simulink model "altitude_controller_design_harness"  (R2025b)
settings: Solver=VariableStepAuto  StartTime=0.0  StopTime=5  RelTol=1e-3
InitFcn:
  | currentControllerInit;
  | controller_mode = controller_modes.PRESSURE
  | 
  | fluid_constants;
  | plant_parameters;
undefined symbols (not defined in the file or in its folder): c_d, controller_modes, controllerGains, DiscIntNeverNeededParam, fluid, mass, nozzle_diameter, X0
libraries: simulink x7, metux_library x5, eeGeneralControl x4, simulink_extras x2, slpidlib x1
settings Model: DataDictionary=motorData.sldd  Creator=karadeli  LastModifiedBy=90507
settings DebuggingCC: ParamSuppressDoubleToSinglePrecisionLossMsg=on

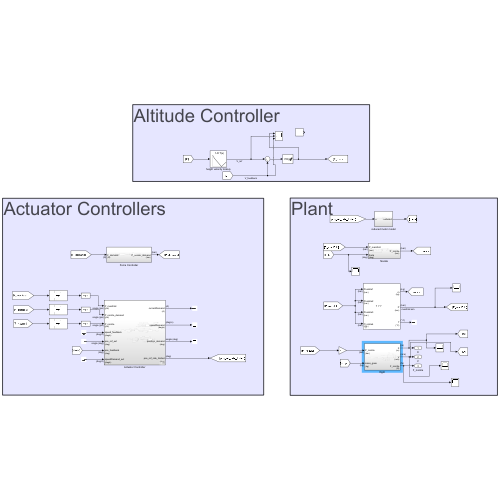
[thumbnail: Simulink's stored preview of the top-level diagram]
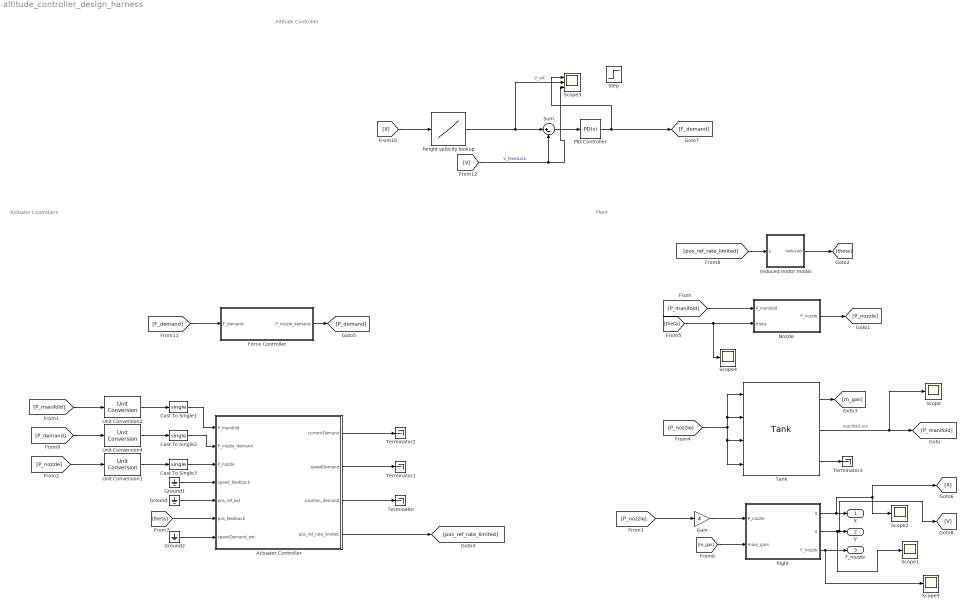
== system altitude_controller_design_harness ==
  note: Altitude Controller
  note: Actuator Controllers
  note: Plant
  Actuator Controller : Subsystem
  Cast To Single1 : DataTypeConversion  OutDataTypeStr=single  SaturateOnIntegerOverflow=off  RndMeth=Floor
  Cast To Single2 : DataTypeConversion  OutDataTypeStr=single  SaturateOnIntegerOverflow=off  RndMeth=Floor
  Cast To Single3 : DataTypeConversion  OutDataTypeStr=single  SaturateOnIntegerOverflow=off  RndMeth=Floor
  Force Controller : Subsystem
  Gain : Gain  Gain=4
  Ground : Ground
  Ground1 : Ground
  Ground2 : Ground
  Nozzle : Subsystem
  PID Controller : slpidlib/PID Controller  Controller=PD  Form=Parallel  TimeDomain=Continuous-time  UseExternalTs=off  SampleTime=-1  IntegratorMethod=Forward Euler  FilterMethod=Forward Euler  ControllerParametersSource=internal  P=180  I=1  UseKiTs=off  D=0  UseExternalDerivativeSource=off  N=100  UseFilter=on  TunerSelectOption=Transfer Function Based (PID Tuner App)  InitialConditionSource=internal  InitialConditionForIntegrator=0  InitialConditionForFilter=0  DifferentiatorICPrevScaledInput=0  ExternalReset=none  TrackingMode=off  Kt=1  LimitOutput=on  SatLimitsSource=internal  UpperSaturationLimit=inf  LowerSaturationLimit=0  LinearizeAsGain=on  AntiWindupMode=none  Kb=1  LimitIntegrator=off  UpperIntegratorSaturationLimit=inf  LowerIntegratorSaturationLimit=-inf  POutMin=[]  POutMax=[]  IOutMin=[]  IOutMax=[]  DOutMin=[]  DOutMax=[]  NOutMin=[]  NOutMax=[]  SumOutMin=[]  SumOutMax=[]  SaturationOutMin=[]  SaturationOutMax=[]  PParamMin=[]  PParamMax=[]  IParamMin=[]  IParamMax=[]  DParamMin=[]  DParamMax=[]  NParamMin=[]  NParamMax=[]  KbParamMin=[]  KbParamMax=[]  KtParamMin=[]  KtParamMax=[]  KbOutMin=[]  KbOutMax=[]  KtOutMin=[]  KtOutMax=[]  IntegratorOutMin=[]  IntegratorOutMax=[]  FilterOutMin=[]  FilterOutMax=[]  SumI1OutMin=[]  SumI1OutMax=[]  SumI2OutMin=[]  SumI2OutMax=[]  SumI3OutMin=[]  SumI3OutMax=[]  SumI4OutMin=[]  SumI4OutMax=[]  SumDOutMin=[]  SumDOutMax=[]  DifferentiatorOutMin=[]  DifferentiatorOutMax=[]  FilterDiffOutCoefMin=[]  FilterDiffOutCoefMax=[]  ReciprocalOutMin=[]  ReciprocalOutMax=[]  SumDenOutMin=[]  SumDenOutMax=[]  SumNumOutMin=[]  SumNumOutMax=[]  DivideOutMin=[]  DivideOutMax=[]  UdiffTsProdOutMin=[]  UdiffTsProdOutMax=[]  NTsProdOutMin=[]  NTsProdOutMax=[]  UintegralTsProdOutMin=[]  UintegralTsProdOutMax=[]  UngainTsProdOutMin=[]  UngainTsProdOutMax=[]  ClampingZeroOutDataTypeStr=Inherit: Inherit via back propagation  ClampingZeroOutMin=[]  ClampingZeroOutMax=[]  FilterDenConstantOutDataTypeStr=Inherit: Inherit via back propagation  FilterDenConstantOutMin=[]  FilterDenConstantOutMax=[]  PCopyOutDataTypeStr=Inherit: Inherit via back propagation  PCopyOutMin=[]  PCopyOutMax=[]  NCopyOutDataTypeStr=Inherit: Inherit via back propagation  NCopyOutMin=[]  NCopyOutMax=[]  IntegratorContinuousStateAttributes=''  IntegratorStateMustResolveToSignalObject=off  IntegratorRTWStateStorageClass=Auto  FilterContinuousStateAttributes=''  FilterStateMustResolveToSignalObject=off  FilterRTWStateStorageClass=Auto  ParallelPVariant=InternalParameters  IdealPVariant=Disabled  IVariant=Disabled  DVariant=InternalParameters  IntegratorVariant=Disabled  SatVariant=Enabled  AWVariant=Disabled  PCopyVariant=Disabled  TRVariant=Disabled  FdbkBlocksVariant=Forward  IdealPFdbkVariant=Disabled  SatFdbkVariant=Disabled  DerivativeFilterVariant=ContFilter  NVariant=InternalParameters  NCopyVariant=Disabled  FilterICVariant=InternalICsFilter  IntegratorICVariant=Disabled  ExternalResetVariant=Disabled  TRSumVariant=Passthrough  SumFdbkVariant=Disabled  SumVariant=Sum_PD  TsampFilterVariant=InternalTs  TsampNgainVariant=Passthrough  TsampIntegralVariant=Disabled_SignalSpec  ExternalSaturationOutDataTypeStr=Inherit: Same as second input  DerivativeSourceVariant=ErrorSignal  PreIntVariant=InternalPreInt
  Scope{,1..2,4..5} (5 alike) : Scope
      Scope settings: ActiveDisplayYMinimum=-1  ActiveDisplayYMaximum=1  DataLoggingVariableName=ScopeData12
      Scope1 settings: ActiveDisplayYMinimum=-12.245566347072526  ActiveDisplayYMaximum=6.6093021776689689  DataLoggingVariableName=ScopeData13
      Scope2 settings: ActiveDisplayYMinimum=-1.1324371537865316  ActiveDisplayYMaximum=10.125826350420725  DataLoggingVariableName=ScopeData14
      Scope4 settings: ActiveDisplayYMinimum=-135.02216749767223  ActiveDisplayYMaximum=1215.1995074790502  DataLoggingVariableName=ScopeData24
      Scope5 settings: ActiveDisplayYMinimum=-1  ActiveDisplayYMaximum=1  DataLoggingVariableName=ScopeData25
  Scope3 : Scope  NumInputPorts=3
      settings: ActiveDisplayYMinimum=-1  ActiveDisplayYMaximum=1  DataLoggingVariableName=ScopeData15
  Step : Step  Time=0.75  After=180  SampleTime=0
  Sum : Sum  Inputs=|+-
  Tank : metux_library/Tank  P0=300  T0=40  mdotGain=fluid.mdotGain  V=fluid.V  R=fluid.R  Cv=fluid.Cv  Patm=fluid.Patm
  Terminator{,1..3} (4 alike) : Terminator
  Unit Conversion1 : UnitConversion
  Unit Conversion2 : UnitConversion
  Unit Conversion4 : UnitConversion
  flight : Subsystem
  height velocity lookup : Lookup_n-D  NumberOfTableDimensions=1  BreakpointsForDimension1=[0 1 6 9]  Table=[0 -2 -8 -5]  InternalRulePriority=Speed  RndMeth=Simplest
  reduced motor model : Subsystem
  X : Outport
  V : Outport  Port=2
  F_nozzle : Outport  Port=3
  wires:
  flight/2(V) -> Scope1/1, [V], V/1
  flight/3(F_nozzle) -> Scope5/1, F_nozzle/1
  flight/1(X) -> [X], Scope2/1, X/1
  [theta] -> Scope4/1, Nozzle/2(theta)
  Tank/2 -> [P_manifold], Scope/1  "manifold sim"
  [P_manifold] -> Unit Conversion2/1
  Actuator Controller/3(position_demand) -> Terminator/1
  Actuator Controller/2(speedDemand) -> Terminator1/1
  Actuator Controller/1(currentDemand) -> Terminator2/1
  Ground/1 -> Actuator Controller/5(pos_ref_ext)
  Tank/1 -> [m_gas]
  [m_gas] -> flight/2(mass_gass)
  Tank/3 -> Terminator3/1
  reduced motor model/1(reduced) -> [theta]
  [theta] -> Actuator Controller/6(pos_feedback)
  [pos_ref_rate_limited] -> reduced motor model/1(u)
  Cast To Single2/1 -> Actuator Controller/2(P_nozzle_demand)
  Ground1/1 -> Actuator Controller/4(speed_feedback)
  Ground2/1 -> Actuator Controller/7(speedDemand_ext)
  [P_nozzle] -> Tank/1, Tank/2, Tank/4, Tank/3
  Nozzle/1(P_nozzle) -> [P_nozzle]
  Unit Conversion4/1 -> Cast To Single2/1
  [P_manifold] -> Nozzle/1(P_manifold)
  Unit Conversion1/1 -> Cast To Single3/1
  [P_nozzle] -> Gain/1
  [P_nozzle] -> Unit Conversion1/1
  Cast To Single3/1 -> Actuator Controller/3(P_nozzle)
  Unit Conversion2/1 -> Cast To Single1/1
  Cast To Single1/1 -> Actuator Controller/1(P_manifold)
  Force Controller/1(P_nozzle_demand) -> [P_demand]
  [P_demand] -> Unit Conversion4/1
  Actuator Controller/4(pos_ref_rate_limited) -> [pos_ref_rate_limited]
  Sum/1 -> PID Controller/1
  PID Controller/1 -> Scope3/1, [F_demand]
  [F_demand] -> Force Controller/1(F_demand)
  height velocity lookup/1 -> Scope3/2, Sum/1  "V_ref"
  [X] -> height velocity lookup/1
  [V] -> Scope3/3, Sum/2  "V_feedback"
  Gain/1 -> flight/1(P_nozzle)

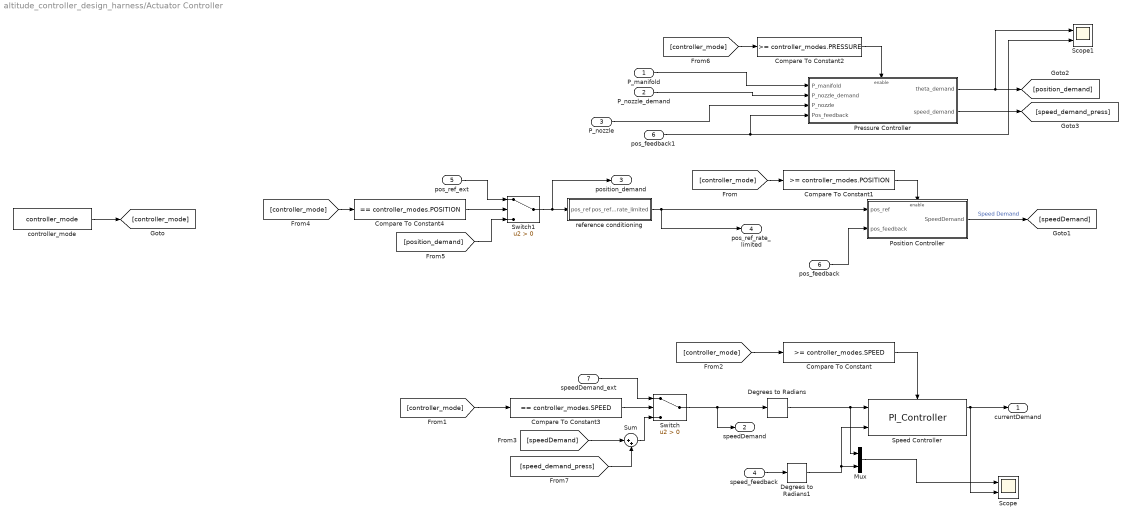
== system altitude_controller_design_harness/Actuator Controller ==
  P_manifold : Inport  OutDataTypeStr=single  Unit=psi  PortDimensions=1  SampleTime=1/1000
  P_nozzle_demand : Inport  Port=2  OutDataTypeStr=single  Unit=psi  PortDimensions=1  SampleTime=1/1000
  P_nozzle : Inport  Port=3  OutDataTypeStr=single  Unit=psi  PortDimensions=1  SampleTime=1/1000
  speed_feedback : Inport  Port=4  Unit=deg/s  SampleTime=controllerGains.speed.Ts  Interpolate=off
  pos_ref_ext : Inport  Port=5  OutDataTypeStr=single  Unit=deg  SampleTime=controllerGains.position.Ts  Interpolate=off
  pos_feedback : Inport  Port=6  Unit=deg  SampleTime=controllerGains.position.Ts  Interpolate=off
  speedDemand_ext : Inport  Port=7  Unit=deg/s
  Compare To Constant : simulink/Logic and Bit Operations/Compare To Constant  relop=>=  const=controller_modes.SPEED  OutDataTypeStr=boolean
  Compare To Constant1 : simulink/Logic and Bit Operations/Compare To Constant  relop=>=  const=controller_modes.POSITION  OutDataTypeStr=boolean
  Compare To Constant2 : simulink/Logic and Bit Operations/Compare To Constant  relop=>=  const=controller_modes.PRESSURE  OutDataTypeStr=boolean
  Compare To Constant3 : simulink/Logic and Bit Operations/Compare To Constant  relop===  const=controller_modes.SPEED  OutDataTypeStr=boolean
  Compare To Constant4 : simulink/Logic and Bit Operations/Compare To Constant  relop===  const=controller_modes.POSITION  OutDataTypeStr=boolean
  Degrees to Radians : simulink_extras/Transformations/Degrees to Radians
  Degrees to Radians1 : simulink_extras/Transformations/Degrees to Radians
  Mux : Mux  Inputs=2
  Position Controller : Subsystem
  Pressure Controller : Subsystem
  Scope : Scope  NumInputPorts=2
      settings: ActiveDisplayYMinimum=-3482.2818450927725  ActiveDisplayYMaximum=28164.697982788086
  Scope1 : Scope  NumInputPorts=2
      settings: ActiveDisplayYMinimum=-329.76221466064453  ActiveDisplayYMaximum=370.11640167236328
  Speed Controller : metux_library/PI_Controller  Kp=controllerGains.speed.Kp  Ki=controllerGains.speed.Ki  SatMax=controllerGains.speed.SatMax  SatMin=controllerGains.speed.SatMin  Ts=controllerGains.speed.Ts  RateLimiterMax=controllerGains.speed.RateLimiterMax  RateLimiterMin=controllerGains.speed.RateLimiterMin
  Sum : Sum  Inputs=|++
  Switch : Switch  Criteria=u2 > Threshold  SaturateOnIntegerOverflow=off  InputSameDT=off
  Switch1 : Switch  Criteria=u2 > Threshold  SaturateOnIntegerOverflow=off  InputSameDT=off
  controller_mode : Constant  Value=controller_mode  SampleTime=-1
  pos_feedback1 : InportShadow  Port=6  Unit=deg  SampleTime=controllerGains.position.Ts  Interpolate=off
  reference conditioning : Subsystem
  currentDemand : Outport  Unit=A
  speedDemand : Outport  Port=2  Unit=deg/s
  position_demand : Outport  Port=3  OutDataTypeStr=single  Unit=deg
  pos_ref_rate_limited : Outport  Port=4  Unit=deg  SampleTime=1/1000
  wires:
  Pressure Controller/1(theta_demand) -> [position_demand], Scope1/1
  P_nozzle_demand/1 -> Pressure Controller/2(P_nozzle_demand)
  [controller_mode] -> Compare To Constant4/1
  controller_mode/1 -> [controller_mode]
  speedDemand_ext/1 -> Switch/1
  Mux/1 -> Scope/1
  Sum/1 -> Switch/3
  speed_feedback/1 -> Degrees to Radians1/1
  Position Controller/1(SpeedDemand) -> [speedDemand]  "Speed Demand"
  Degrees to Radians/1 -> Mux/1, Speed Controller/1
  Switch/1 -> speedDemand/1, Degrees to Radians/1
  Compare To Constant1/1 -> Position Controller/Enable
  [controller_mode] -> Compare To Constant2/1
  Compare To Constant/1 -> Speed Controller/Enable
  pos_feedback/1 -> Position Controller/2(pos_feedback)
  Compare To Constant2/1 -> Pressure Controller/Enable
  P_nozzle/1 -> Pressure Controller/3(P_nozzle)
  Compare To Constant4/1 -> Switch1/2
  [position_demand] -> Switch1/3
  [controller_mode] -> Compare To Constant1/1
  Speed Controller/1 -> currentDemand/1, Scope/2
  [controller_mode] -> Compare To Constant/1
  P_manifold/1 -> Pressure Controller/1(P_manifold)
  pos_ref_ext/1 -> Switch1/1
  Switch1/1 -> position_demand/1, reference conditioning/1(pos_ref)
  Degrees to Radians1/1 -> Speed Controller/2, Mux/2
  [controller_mode] -> Compare To Constant3/1
  Compare To Constant3/1 -> Switch/2
  reference conditioning/1(pos_ref_rate_limited) -> pos_ref_rate_limited/1, Position Controller/1(pos_ref)
  pos_feedback1/1 -> Pressure Controller/4(Pos_feedback), Scope1/2
  Pressure Controller/2(speed_demand) -> [speed_demand_press]
  [speedDemand] -> Sum/1
  [speed_demand_press] -> Sum/2

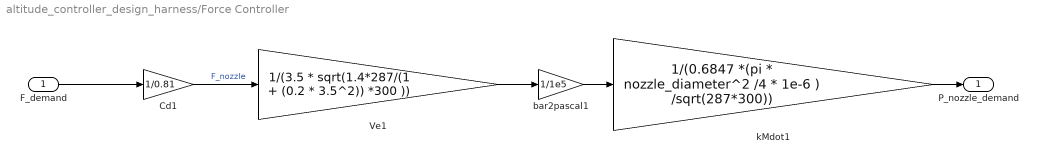
== system altitude_controller_design_harness/Force Controller ==
  F_demand : Inport  Unit=N  SampleTime=1/1000
  Cd1 : Gain  Gain=1/0.81
  Ve1 : Gain  Gain=1/(3.5 * sqrt(1.4*287/(1 + (0.2 * 3.5^2)) *300 ))
  bar2pascal1 : Gain  Gain=1/1e5
  kMdot1 : Gain  Gain=1/(0.6847 *(pi * nozzle_diameter^2 /4 * 1e-6 ) /sqrt(287*300))
  P_nozzle_demand : Outport  Unit=bar  SampleTime=1/1000
  wires:
  kMdot1/1 -> P_nozzle_demand/1
  bar2pascal1/1 -> kMdot1/1
  Ve1/1 -> bar2pascal1/1
  Cd1/1 -> Ve1/1  "F_nozzle"
  F_demand/1 -> Cd1/1

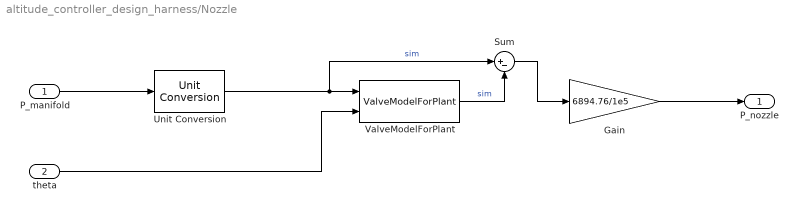
== system altitude_controller_design_harness/Nozzle ==
  P_manifold : Inport  Unit=bar
  theta : Inport  Port=2  Unit=deg
  Gain : Gain  Gain=6894.76/1e5
  Sum : Sum  Inputs=|+-
  Unit Conversion : UnitConversion
  ValveModelForPlant : metux_library/ValveModelForPlant  C_max=0.9197  alpha=51.8534
  P_nozzle : Outport  Unit=bar
  wires:
  theta/1 -> ValveModelForPlant/2
  P_manifold/1 -> Unit Conversion/1
  Sum/1 -> Gain/1
  ValveModelForPlant/1 -> Sum/2  "sim"
  Gain/1 -> P_nozzle/1
  Unit Conversion/1 -> Sum/1, ValveModelForPlant/1  "sim"

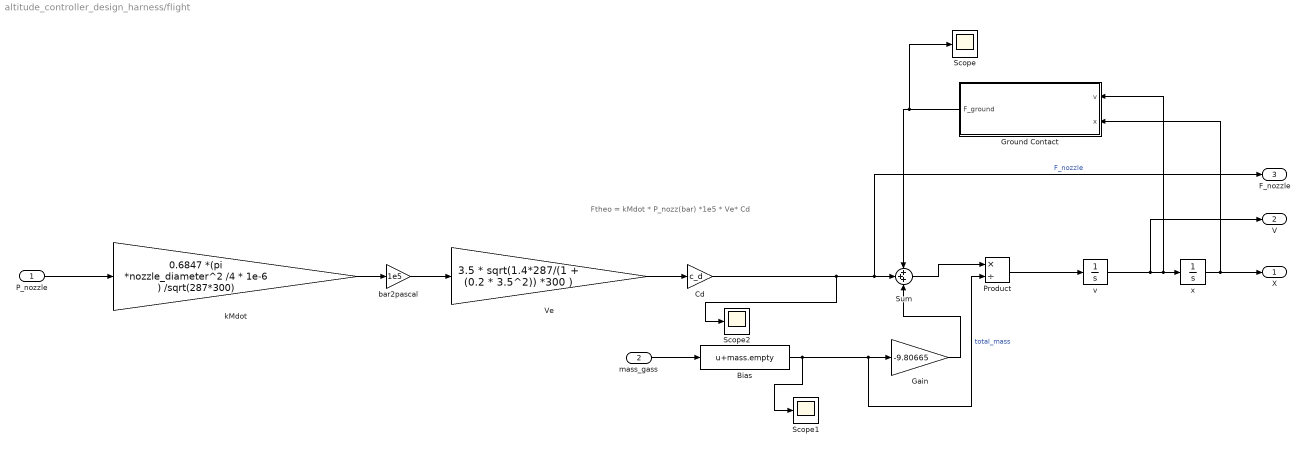
== system altitude_controller_design_harness/flight ==
  note: Ftheo = kMdot * P_nozz(bar) *1e5 * Ve* Cd
  P_nozzle : Inport  Unit=bar
  mass_gass : Inport  Port=2  Unit=kg
  Bias : Bias  Bias=mass.empty  SaturateOnIntegerOverflow=off
  Cd : Gain  Gain=c_d
  Gain : Gain  Gain=-9.80665
  Ground Contact : Subsystem
  Product : Product  Inputs=*/
  Scope : Scope
      settings: ActiveDisplayYMinimum=-179.96473711218755  ActiveDisplayYMaximum=786.35837452552653  DataLoggingVariableName=ScopeData19
  Scope1 : Scope
      settings: ActiveDisplayYMinimum=-1  ActiveDisplayYMaximum=1  DataLoggingVariableName=ScopeData20
  Scope2 : Scope
      settings: ActiveDisplayYMinimum=-1  ActiveDisplayYMaximum=1  DataLoggingVariableName=ScopeData21
  Sum : Sum  Inputs=+++
  Ve : Gain  Gain=3.5 * sqrt(1.4*287/(1 + (0.2 * 3.5^2)) *300 )
  bar2pascal : Gain  Gain=1e5
  kMdot : Gain  Gain=0.6847 *(pi *nozzle_diameter^2 /4 * 1e-6 ) /sqrt(287*300)
  v : Integrator
  x : Integrator  InitialCondition=X0
  X : Outport  Unit=m
  V : Outport  Port=2  Unit=m/s
  F_nozzle : Outport  Port=3  Unit=N
  wires:
  Gain/1 -> Sum/3
  Sum/1 -> Product/1
  x/1 -> Ground Contact/2(x), X/1
  kMdot/1 -> bar2pascal/1
  Bias/1 -> Scope1/1, Product/2, Gain/1  "total_mass"
  bar2pascal/1 -> Ve/1
  Cd/1 -> Scope2/1, F_nozzle/1, Sum/2  "F_nozzle"
  Product/1 -> v/1
  Ve/1 -> Cd/1
  P_nozzle/1 -> kMdot/1
  mass_gass/1 -> Bias/1
  v/1 -> Ground Contact/1(v), x/1, V/1
  Ground Contact/1(F_ground) -> Scope/1, Sum/1

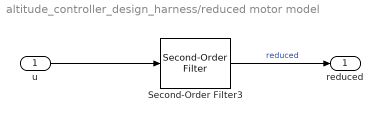
== system altitude_controller_design_harness/reduced motor model ==
  u : Inport
  Second-Order Filter3 : eeGeneralControl/Second-Order Filter  FilterType=Low-pass  fn=21.64  Zeta=0.86  Ts=-1  A0=0  Ph0=0  f0=0  b0=0
      settings: LibrarySourceBlock=ee_sl_lib/General Control/Second-Order Filter
  reduced : Outport
  wires:
  Second-Order Filter3/1 -> reduced/1  "reduced"
  u/1 -> Second-Order Filter3/1

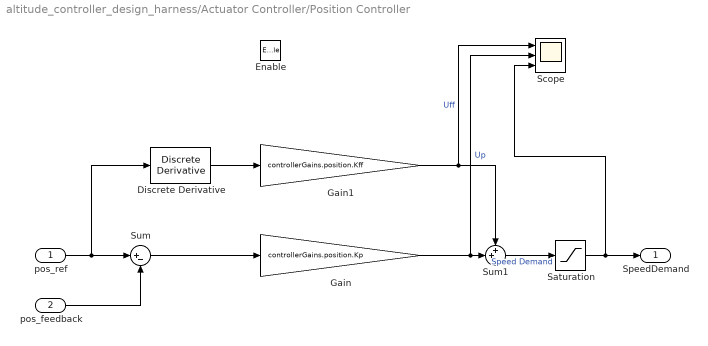
== system altitude_controller_design_harness/Actuator Controller/Position Controller ==
  pos_ref : Inport  Unit=deg
  pos_feedback : Inport  Port=2  Unit=deg
  Enable : EnablePort  StatesWhenEnabling=reset
  Discrete Derivative : simulink/Discrete/Discrete Derivative  gainval=1.0  ICPrevScaledInput=0.0  OutMin=[]  OutMax=[]  OutDataType=fixdt(1, 16)  OutScaling=2^-10  DoSatur=off
  Gain : Gain  Gain=controllerGains.position.Kp
  Gain1 : Gain  Gain=controllerGains.position.Kff
  Saturation : Saturate  UpperLimit=controllerGains.position.SatMax  LowerLimit=controllerGains.position.SatMin
  Scope : Scope  NumInputPorts=3
      settings: ActiveDisplayYMinimum=-3294.8933715820312  ActiveDisplayYMaximum=3471.4622192382812
  Sum : Sum  Inputs=|+-
  Sum1 : Sum  Inputs=++|
  SpeedDemand : Outport  Unit=deg/s  OutputWhenDisabled=reset  InitialOutput=[0.0]
  wires:
  Saturation/1 -> Scope/3, SpeedDemand/1
  pos_feedback/1 -> Sum/2
  Gain/1 -> Scope/2, Sum1/2  "Up"
  Sum/1 -> Gain/1
  pos_ref/1 -> Discrete Derivative/1, Sum/1
  Sum1/1 -> Saturation/1  "Speed Demand"
  Discrete Derivative/1 -> Gain1/1
  Gain1/1 -> Scope/1, Sum1/1  "Uff"

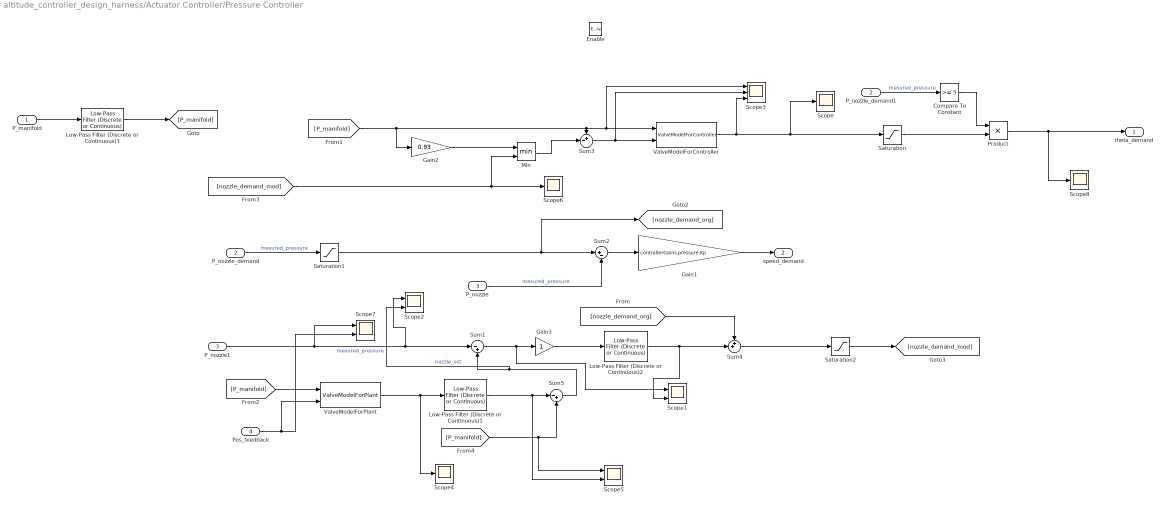
== system altitude_controller_design_harness/Actuator Controller/Pressure Controller ==
  P_manifold : Inport
  P_nozzle_demand : Inport  Port=2
  P_nozzle : Inport  Port=3
  Pos_feedback : Inport  Port=4
  Enable : EnablePort  StatesWhenEnabling=reset
  Compare To Constant : simulink/Logic and Bit Operations/Compare To Constant  relop=>=  const=5  OutDataTypeStr=boolean
  Gain1 : Gain  Gain=controllerGains.pressure.Kp
  Gain2 : Gain  Gain=0.93
  Gain3 : Gain
  Low-Pass Filter (Discrete or Continuous)1 : eeGeneralControl/Low-Pass Filter (Discrete or Continuous)  K=1  T=0.001  B=inf  A=-inf  init_option=Inherited from block input  x0=0  Ts=-1
  Low-Pass Filter (Discrete or Continuous)2 : eeGeneralControl/Low-Pass Filter (Discrete or Continuous)  K=1  T=0.004  B=250  A=-250  init_option=Inherited from block input  x0=0  Ts=-1
  Low-Pass Filter (Discrete or Continuous)3 : eeGeneralControl/Low-Pass Filter (Discrete or Continuous)  K=single(1)  T=single(0.005)  B=inf  A=-inf  init_option=Inherited from block input  x0=0  Ts=-1
  Min : MinMax  Inputs=2
  P_nozzle1 : InportShadow  Port=3
  P_nozzle_demand1 : InportShadow  Port=2
  Product : Product
  Saturation : Saturate  UpperLimit=1080  LowerLimit=0
  Saturation1 : Saturate  UpperLimit=4000  LowerLimit=0
  Saturation2 : Saturate  UpperLimit=4000  LowerLimit=0
  Scope{,4,6,8} (4 alike) : Scope
      Scope settings: ActiveDisplayYMinimum=-15.395192146301266  ActiveDisplayYMaximum=138.55672931671143  DataLoggingVariableName=ScopeData2
      Scope4 settings: ActiveDisplayYMinimum=1007.1971893310547  ActiveDisplayYMaximum=2357.6605987548828  DataLoggingVariableName=ScopeData6
      Scope6 settings: ActiveDisplayYMinimum=-112.49999999999997  ActiveDisplayYMaximum=1012.5  DataLoggingVariableName=ScopeData8
      Scope8 settings: ActiveDisplayYMinimum=-18.167575836181637  ActiveDisplayYMaximum=163.50818252563477  DataLoggingVariableName=ScopeData10
  Scope{1..2,5,7} (4 alike) : Scope  NumInputPorts=2
      Scope1 settings: ActiveDisplayYMinimum=16.466037750244148  ActiveDisplayYMaximum=359.39812850952148  DataLoggingVariableName=ScopeData4
      Scope2 settings: ActiveDisplayYMinimum=-179.26073789596555  ActiveDisplayYMaximum=1025.8466792106628  DataLoggingVariableName=ScopeData5
      Scope5 settings: ActiveDisplayYMinimum=1218.2213745117188  ActiveDisplayYMaximum=2587.3870239257812  DataLoggingVariableName=ScopeData7
      Scope7 settings: ActiveDisplayYMinimum=-62.757351875305176  ActiveDisplayYMaximum=64.080883979797363  DataLoggingVariableName=ScopeData9
  Scope3 : Scope  NumInputPorts=3
      settings: ActiveDisplayYMinimum=-431.94372558593739  ActiveDisplayYMaximum=3887.4935302734375  DataLoggingVariableName=ScopeData3
  Sum1 : Sum  Inputs=|-+
  Sum2 : Sum  Inputs=|+-
  Sum3 : Sum  Inputs=+-|  OutDataTypeStr=single
  Sum4 : Sum  Inputs=++|
  Sum5 : Sum  Inputs=|-+
  ValveModelForController : metux_library/ValveModelForController  alpha=51.8534  C_max=0.9197
  ValveModelForPlant : metux_library/ValveModelForPlant  C_max=0.9197  alpha=51.8534
  theta_demand : Outport  OutputWhenDisabled=reset  InitialOutput=0
  speed_demand : Outport  Port=2  OutputWhenDisabled=reset  InitialOutput=0
  wires:
  Saturation/1 -> Product/2
  Compare To Constant/1 -> Product/1
  P_nozzle_demand1/1 -> Compare To Constant/1  "mesured_pressure"
  Saturation2/1 -> [nozzle_demand_mod]
  Saturation1/1 -> [nozzle_demand_org], Sum2/1
  Sum1/1 -> Gain3/1, Scope1/1
  Product/1 -> theta_demand/1, Scope8/1
  Gain2/1 -> Min/1
  P_manifold/1 -> Low-Pass Filter (Discrete or Continuous)3/1
  P_nozzle_demand/1 -> Saturation1/1  "mesured_pressure"
  Sum3/1 -> Scope3/2, ValveModelForController/2
  P_nozzle/1 -> Sum2/2  "mesured_pressure"
  Gain1/1 -> speed_demand/1
  ValveModelForController/1 -> Scope3/3, Saturation/1, Scope/1
  Sum2/1 -> Gain1/1
  ValveModelForPlant/1 -> Low-Pass Filter (Discrete or Continuous)1/1, Scope4/1
  Sum5/1 -> Sum1/2, Scope2/2  "nozzle_est"
  [nozzle_demand_org] -> Sum4/1
  [P_manifold] -> Sum5/2, Scope5/1
  Sum4/1 -> Saturation2/1
  [nozzle_demand_mod] -> Scope6/1, Min/2
  Min/1 -> Sum3/2
  Gain3/1 -> Low-Pass Filter (Discrete or Continuous)2/1
  Pos_feedback/1 -> ValveModelForPlant/2, Scope7/2
  [P_manifold] -> ValveModelForPlant/1
  [P_manifold] -> Sum3/1, Scope3/1, ValveModelForController/1, Gain2/1
  Low-Pass Filter (Discrete or Continuous)1/1 -> Sum5/1, Scope5/2
  P_nozzle1/1 -> Sum1/1, Scope2/1, Scope7/1  "mesured_pressure"
  Low-Pass Filter (Discrete or Continuous)3/1 -> [P_manifold]
  Low-Pass Filter (Discrete or Continuous)2/1 -> Sum4/2, Scope1/2

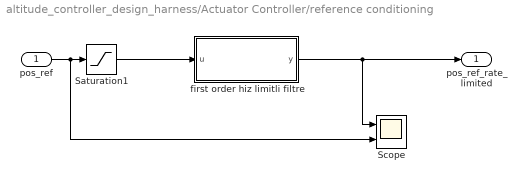
== system altitude_controller_design_harness/Actuator Controller/reference conditioning ==
  pos_ref : Inport
  Saturation1 : Saturate  UpperLimit=360*4  LowerLimit=0
  Scope : Scope  NumInputPorts=2
      settings: ActiveDisplayYMinimum=115.37295030320635  ActiveDisplayYMaximum=137.10329135900082  DataLoggingVariableName=ScopeData11
  first order hiz limitli filtre : Subsystem
  pos_ref_rate_limited : Outport
  wires:
  pos_ref/1 -> Saturation1/1, Scope/2
  Saturation1/1 -> first order hiz limitli filtre/1(u)
  first order hiz limitli filtre/1(y) -> pos_ref_rate_limited/1, Scope/1

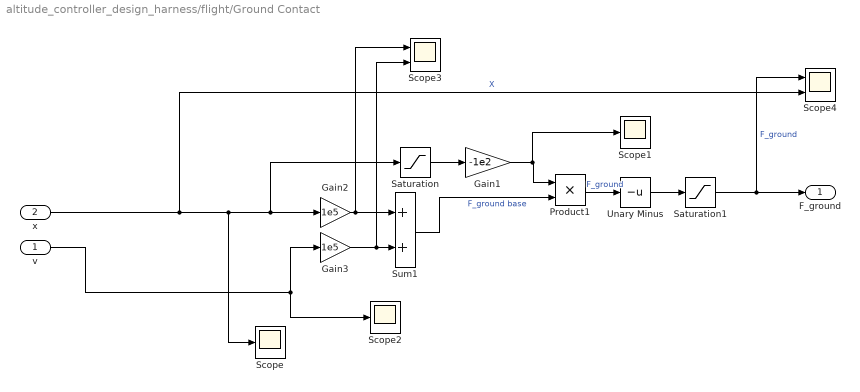
== system altitude_controller_design_harness/flight/Ground Contact ==
  v : Inport
  x : Inport  Port=2
  Gain1 : Gain  Gain=-1e2
  Gain2 : Gain  Gain=1e5
  Gain3 : Gain  Gain=1e5
  Product1 : Product
  Saturation : Saturate  UpperLimit=0  LowerLimit=-1e-2
  Saturation1 : Saturate  UpperLimit=inf  LowerLimit=0
  Scope : Scope
      settings: ActiveDisplayYMinimum=-0.00064624515579334257  ActiveDisplayYMaximum=7.1805017310371379E-5  DataLoggingVariableName=ScopeData16
  Scope1 : Scope
      settings: ActiveDisplayYMinimum=-0.12499999999999997  ActiveDisplayYMaximum=1.125  DataLoggingVariableName=ScopeData17
  Scope2 : Scope
      settings: ActiveDisplayYMinimum=-12.240152608908808  ActiveDisplayYMaximum=6.6047525948989225  DataLoggingVariableName=ScopeData18
  Scope3 : Scope  NumInputPorts=2
      settings: ActiveDisplayYMinimum=-53205.273508852  ActiveDisplayYMaximum=73840.874785199179  DataLoggingVariableName=ScopeData22
  Scope4 : Scope  NumInputPorts=2
      settings: ActiveDisplayYMinimum=-84.988802031203932  ActiveDisplayYMaximum=501.30945793453066  DataLoggingVariableName=ScopeData23
  Sum1 : Sum
  Unary Minus : UnaryMinus
  F_ground : Outport
  wires:
  Saturation/1 -> Gain1/1
  x/1 -> Scope4/2, Scope/1, Saturation/1, Gain2/1  "X"
  Sum1/1 -> Product1/2  "F_ground base"
  Product1/1 -> Unary Minus/1  "F_ground"
  Gain3/1 -> Scope3/2, Sum1/2
  Gain1/1 -> Scope1/1, Product1/1
  Unary Minus/1 -> Saturation1/1
  Gain2/1 -> Scope3/1, Sum1/1
  Saturation1/1 -> Scope4/1, F_ground/1  "F_ground"
  v/1 -> Gain3/1, Scope2/1

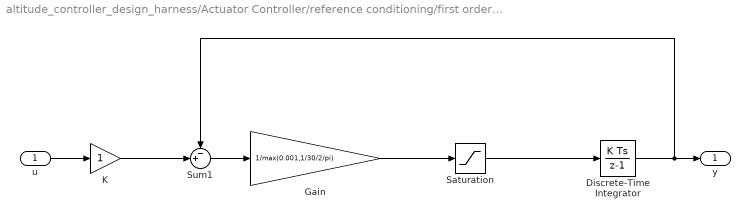
== system altitude_controller_design_harness/Actuator Controller/reference conditioning/first order hiz limitli filtre ==
  u : Inport
  Discrete-Time Integrator : DiscreteIntegrator  SampleTime=-1  ICPrevOutput=DiscIntNeverNeededParam  ICPrevScaledInput=DiscIntNeverNeededParam
  Gain : Gain  Gain=1/max(0.001,1/30/2/pi)
  K : Gain
  Saturation : Saturate  UpperLimit=2400  LowerLimit=-2400
  Sum1 : Sum  Inputs=-+|
  y : Outport  VectorParamsAs1DForOutWhenUnconnected=off
  wires:
  K/1 -> Sum1/2
  Sum1/1 -> Gain/1
  Gain/1 -> Saturation/1
  Discrete-Time Integrator/1 -> Sum1/1, y/1
  u/1 -> K/1
  Saturation/1 -> Discrete-Time Integrator/1
